simulink model "sim_ballAndPlate"  (R2025a)
settings: Solver=FixedStepAuto  StartTime=0.0  StopTime=inf  FixedStep=0.001  RelTol=1e-3
values from neighbouring files (symbols this model uses):
  a = [xddot; yddot]    [generate_circular_trajectory.m]    (also in generate_square_trajectory.m)
  enable = 1    [setParams.m]
  g = 9.81    [MPC_design.m]    (also in MPC_design_condensed.m; MPC_design_realtime.m; compute_mpc_params.m; setParams.m)
  I_max = 3    [setParams.m]
  inner_I_sat = 1    [setParams.m]
  K_lqr = dlqr(Ad, Bd, Q_lqr, R_lqr)    [setParams.m]
  Km = 11    [setParams.m]
  m = m_a + 1/3 * m_p    (= 0.345333333333)    [setParams.m]
  Q_kf = diag([1, 100, 1, 100])    [setParams.m]
  r = 0.17    [angleToPos.m]    (also in generate_circular_trajectory.m = [x; xdot; y; ydot]; generate_square_trajectory.m = [x; xdot; y; ydot])
  R_kf = diag([0.1, 0.1])    [setParams.m]
  Ts_Inner = 0.001    [setParams.m]
  x0 = sdpvar(nx,1)    [MPC_design.m]    (also in MPC_design_condensed.m = sdpvar(nx, 1); setParams.m = [0, 0, 0, 0])
  x_init = 0    [setParams.m]
  x_max = 0.03    [setParams.m]
undefined symbols (not defined in the file or in its folder): DiscIntNeverNeededParam, G_A, G_B, G_C
libraries: mpclib x1
settings Model: Creator=thoma  LastModifiedBy=thoma

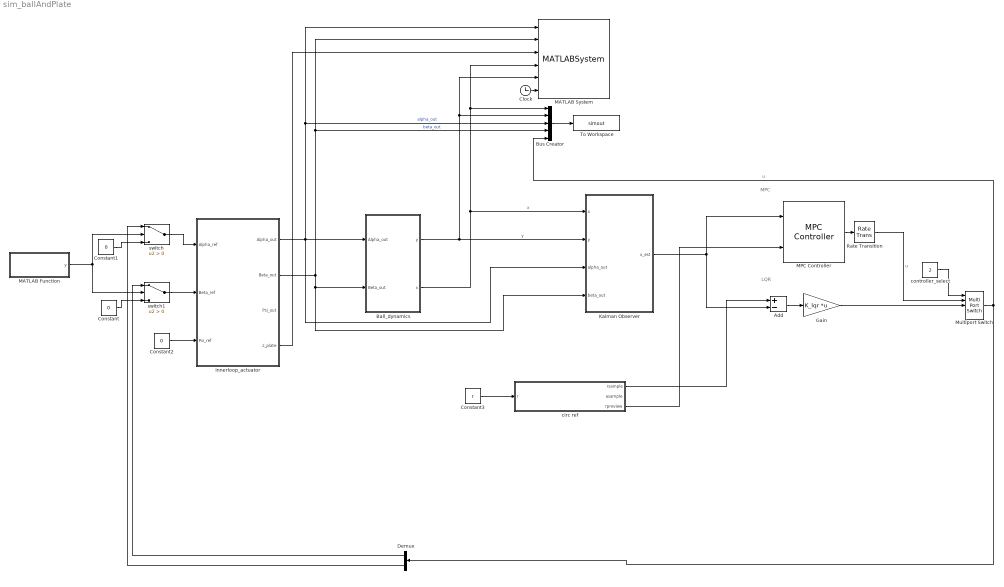
== system sim_ballAndPlate ==
  note: LQR
  note: MPC
  Add : Sum  Inputs=+-
  Ball_dynamics : Subsystem
  Bus Creator : BusCreator  Inputs=5
  Clock : Clock
  Constant : Constant  Value=0
  Constant1 : Constant  Value=0
  Constant2 : Constant  Value=0
  Constant3 : Constant  Value=r
  Demux : Demux  Outputs=2
  Gain : Gain  Gain=K_lqr  Multiplication=Matrix(K*u)
  Innerloop_actuator : Subsystem
  Kalman Observer : Subsystem
  MATLAB Function : MATLAB Function  TreatAsAtomicUnit=on
  MATLAB System : MATLABSystem  System=PlateVisualizer  SimulateUsing=Code generation
      mask Type: PlateVisualizer
  MPC Controller : mpclib/MPC Controller  SCDEnableBlockLinearizationSpecification=on  mpcobj=mpcobj  is_multiple=0  enable_value=0  return_u0=off  updateMPCinCallerWorkspace=on  md_inport=off  mv_inport=off  uref_inport=off  return_cost=off  return_mvseq=off  return_qpstatus=off  return_xseq=off  return_state=off  return_ovseq=off  state_inport=on  umin_inport=off  umax_inport=off  ymin_inport=off  ymax_inport=off  cc_inport=off  ywt_inport=off  uwt_inport=off  duwt_inport=off  rhoeps_inport=off  pm_inport=off  MaximumP=10  HorizonChoice=FixedHorizon  n_ts=0.02  n_p=25  n_mv=2  n_md=0  n_ud=0  n_mo=4  n_uo=0  BlockDataType=double  SampleTimeInherited=off  switch_inport=off
  Multiport Switch : MultiPortSwitch  Inputs=4  SaturateOnIntegerOverflow=off  InputSameDT=off
  Rate Transition : RateTransition
  To Workspace : ToWorkspace  VariableName=simout  SaveFormat=Timeseries  SampleTime=-1
  circ ref : MATLAB Function  TreatAsAtomicUnit=on
  controller_select : Constant  Value=2
  switch : Switch  Criteria=u2 > Threshold  SaturateOnIntegerOverflow=off  InputSameDT=off
  switch1 : Switch  Criteria=u2 > Threshold  SaturateOnIntegerOverflow=off  InputSameDT=off
  wires:
  Constant2/1 -> Innerloop_actuator/3(Psi_ref)
  Innerloop_actuator/2(Beta_out) -> Kalman Observer/4(beta_out), Ball_dynamics/2(Beta_out), Bus Creator/4, MATLAB System/2  "beta_out"
  Innerloop_actuator/1(Alpha_out) -> MATLAB System/1, Bus Creator/3, Kalman Observer/3(alpha_out), Ball_dynamics/1(Alpha_out)  "alpha_out"
  Ball_dynamics/1(y) -> Bus Creator/2, MATLAB System/5, Kalman Observer/2(y)  "y"
  Ball_dynamics/2(x) -> Bus Creator/1, MATLAB System/4, Kalman Observer/1(x)  "x"
  MATLAB Function/1(y) -> switch/2, switch1/2
  Demux/1 -> switch1/1
  switch1/1 -> Innerloop_actuator/2(Beta_ref)
  switch/1 -> Innerloop_actuator/1(Alpha_ref)
  Demux/2 -> switch/1
  Innerloop_actuator/4(z_plate) -> MATLAB System/3
  MPC Controller/1 -> Rate Transition/1
  Multiport Switch/1 -> Demux/1, Bus Creator/5  "u"
  Constant1/1 -> switch/3
  Constant/1 -> switch1/3
  Bus Creator/1 -> To Workspace/1
  Clock/1 -> MATLAB System/6
  circ ref/3(rpreview) -> MPC Controller/2
  Rate Transition/1 -> Multiport Switch/2  "u"
  controller_select/1 -> Multiport Switch/1
  Add/1 -> Gain/1
  circ ref/1(rsample) -> Add/1
  Kalman Observer/1(x_est) -> MPC Controller/1, Add/2
  Gain/1 -> Multiport Switch/3
  Constant3/1 -> circ ref/1(r)

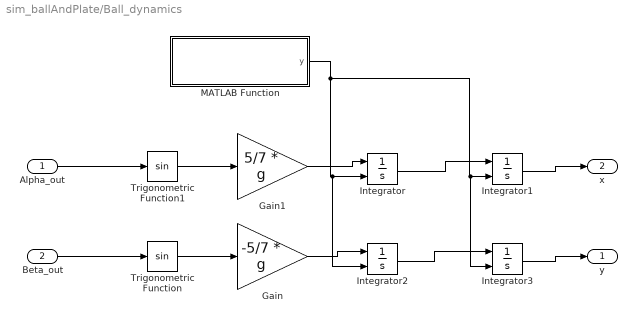
== system sim_ballAndPlate/Ball_dynamics ==
  Alpha_out : Inport
  Beta_out : Inport  Port=2
  Gain : Gain  Gain=-5/7 * g
  Gain1 : Gain  Gain=5/7 * g
  Integrator : Integrator  ExternalReset=rising  InitialCondition=x0(2)
  Integrator1 : Integrator  ExternalReset=rising  InitialCondition=x0(1)
  Integrator2 : Integrator  ExternalReset=rising  InitialCondition=x0(4)
  Integrator3 : Integrator  ExternalReset=rising  InitialCondition=x0(2)
  MATLAB Function : MATLAB Function  TreatAsAtomicUnit=on
  Trigonometric Function : Trigonometry
  Trigonometric Function1 : Trigonometry
  y : Outport
  x : Outport  Port=2
  wires:
  Beta_out/1 -> Trigonometric Function/1
  Trigonometric Function/1 -> Gain/1
  Gain/1 -> Integrator2/1
  Trigonometric Function1/1 -> Gain1/1
  Alpha_out/1 -> Trigonometric Function1/1
  Gain1/1 -> Integrator/1
  Integrator/1 -> Integrator1/1
  Integrator1/1 -> x/1
  Integrator2/1 -> Integrator3/1
  Integrator3/1 -> y/1
  MATLAB Function/1(y) -> Integrator3/2, Integrator1/2, Integrator2/2, Integrator/2

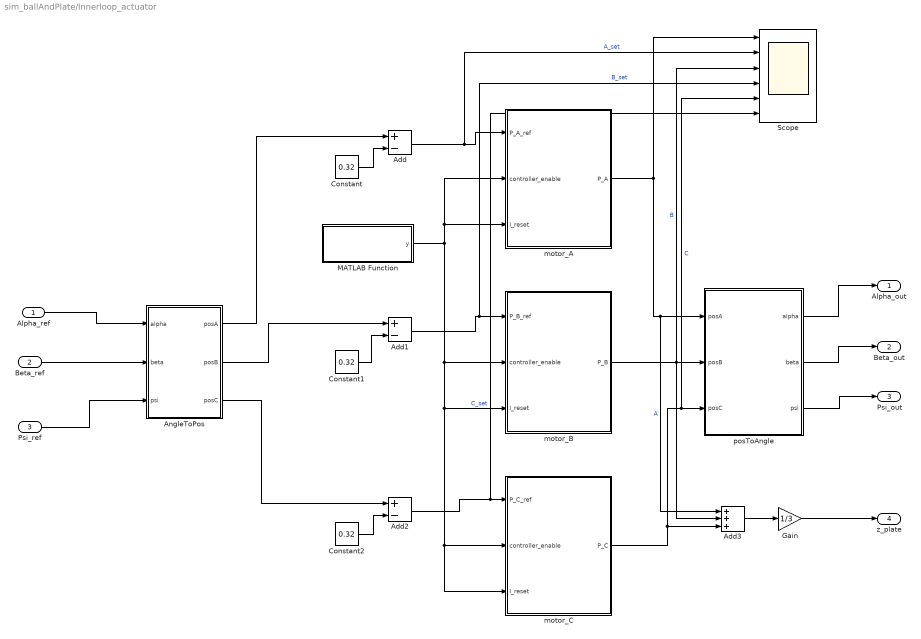
== system sim_ballAndPlate/Innerloop_actuator ==
  Alpha_ref : Inport
  Beta_ref : Inport  Port=2
  Psi_ref : Inport  Port=3
  Add : Sum  Inputs=+-
  Add1 : Sum  Inputs=+-
  Add2 : Sum  Inputs=+-
  Add3 : Sum  Inputs=+++
  "AngleToPos " : MATLAB Function  TreatAsAtomicUnit=on
  Constant : Constant  Value=0.32
  Constant1 : Constant  Value=0.32
  Constant2 : Constant  Value=0.32
  Gain : Gain  Gain=1/3
  MATLAB Function : MATLAB Function  TreatAsAtomicUnit=on
  Scope : Scope  NumInputPorts=6
      settings: ActiveDisplayYMinimum=-0.0017528825710255869  ActiveDisplayYMaximum=0.0020437285369552553
  motor_A : Subsystem
  motor_B : Subsystem
  motor_C : Subsystem
  posToAngle : MATLAB Function  TreatAsAtomicUnit=on
  Alpha_out : Outport
  Beta_out : Outport  Port=2
  Psi_out : Outport  Port=3
  z_plate : Outport  Port=4
  wires:
  Alpha_ref/1 -> "AngleToPos "/1(alpha)
  Beta_ref/1 -> "AngleToPos "/2(beta)
  Psi_ref/1 -> "AngleToPos "/3(psi)
  Constant/1 -> Add/2
  Add/1 -> Scope/2, motor_A/1(P_A_ref)  "A_set"
  motor_A/1(P_A) -> Add3/1, posToAngle/1(posA), Scope/1  "A"
  "AngleToPos "/1(posA) -> Add/1
  posToAngle/1(alpha) -> Alpha_out/1
  "AngleToPos "/2(posB) -> Add1/1
  Add1/1 -> Scope/4, motor_B/1(P_B_ref)  "B_set"
  Constant1/1 -> Add1/2
  "AngleToPos "/3(posC) -> Add2/1
  Add2/1 -> Scope/6, motor_C/1(P_C_ref)  "C_set"
  Constant2/1 -> Add2/2
  motor_C/1(P_C) -> Add3/3, Scope/5, posToAngle/3(posC)  "C"
  motor_B/1(P_B) -> Scope/3, posToAngle/2(posB), Add3/2  "B"
  posToAngle/2(beta) -> Beta_out/1
  posToAngle/3(psi) -> Psi_out/1
  MATLAB Function/1(y) -> motor_B/3(I_reset), motor_C/3(I_reset), motor_C/2(controller_enable), motor_B/2(controller_enable), motor_A/3(I_reset), motor_A/2(controller_enable)
  Add3/1 -> Gain/1
  Gain/1 -> z_plate/1

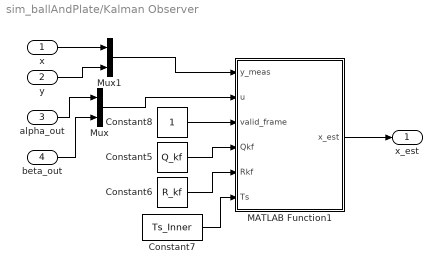
== system sim_ballAndPlate/Kalman Observer ==
  x : Inport
  y : Inport  Port=2
  alpha_out : Inport  Port=3
  beta_out : Inport  Port=4
  Constant5 : Constant  Value=Q_kf
  Constant6 : Constant  Value=R_kf
  Constant7 : Constant  Value=Ts_Inner
  Constant8 : Constant
  MATLAB Function1 : MATLAB Function  TreatAsAtomicUnit=on
  Mux : Mux  Inputs=2
  Mux1 : Mux  Inputs=2
  x_est : Outport
  wires:
  Mux1/1 -> MATLAB Function1/1(y_meas)
  Constant7/1 -> MATLAB Function1/6(Ts)
  Constant5/1 -> MATLAB Function1/4(Qkf)
  x/1 -> Mux1/1
  Mux/1 -> MATLAB Function1/2(u)
  beta_out/1 -> Mux/2
  Constant8/1 -> MATLAB Function1/3(valid_frame)
  Constant6/1 -> MATLAB Function1/5(Rkf)
  MATLAB Function1/1(x_est) -> x_est/1
  y/1 -> Mux1/2
  alpha_out/1 -> Mux/1

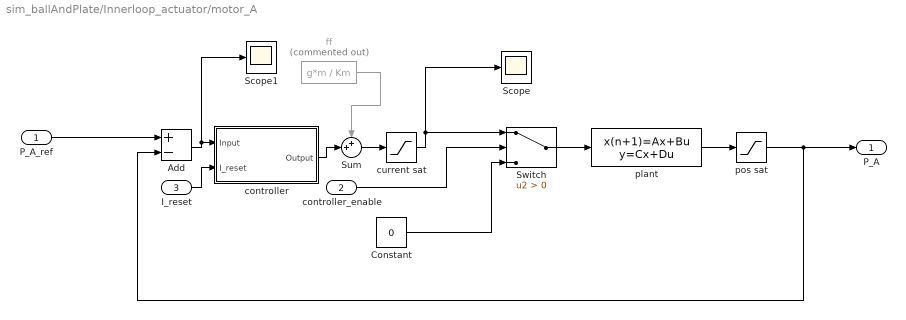
== system sim_ballAndPlate/Innerloop_actuator/motor_A ==
  P_A_ref : Inport
  controller_enable : Inport  Port=2
  I_reset : Inport  Port=3
  Add : Sum  Inputs=+-
  Constant : Constant  Value=0
  Scope : Scope
      settings: ActiveDisplayYMinimum=-0.2151003532733422  ActiveDisplayYMaximum=0.78783772218945147  DataLoggingVariableName=ScopeData3
  Scope1 : Scope
      settings: ActiveDisplayYMinimum=-0.013802200769437761  ActiveDisplayYMaximum=0.022158674956348122  DataLoggingVariableName=ScopeData5
  Sum : Sum  Inputs=++|
  Switch : Switch  Criteria=u2 > Threshold  SaturateOnIntegerOverflow=off  InputSameDT=off
  controller : Subsystem
  current sat : Saturate  UpperLimit=I_max  LowerLimit=-I_max
  ff : Constant  Commented=on  Value=g*m / Km
  plant : DiscreteStateSpace  A=G_A.A  B=G_A.B  C=G_A.C  D=G_A.D  SampleTime=-1
  pos sat : Saturate  UpperLimit=x_max  LowerLimit=-x_max
  P_A : Outport
  wires:
  P_A_ref/1 -> Add/1
  controller/1(Output) -> Sum/2
  plant/1 -> pos sat/1
  pos sat/1 -> Add/2, P_A/1
  controller_enable/1 -> Switch/2
  current sat/1 -> Switch/1, Scope/1
  Switch/1 -> plant/1
  Constant/1 -> Switch/3
  Add/1 -> Scope1/1, controller/1(Input)
  I_reset/1 -> controller/2(I_reset)
  ff/1 -> Sum/1
  Sum/1 -> current sat/1

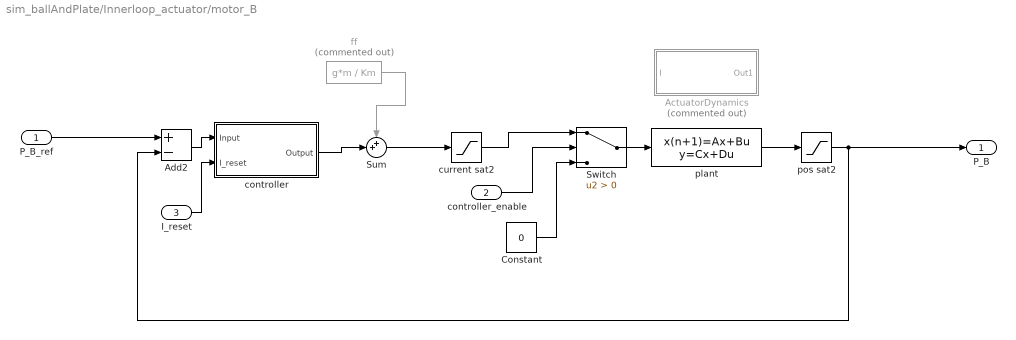
== system sim_ballAndPlate/Innerloop_actuator/motor_B ==
  P_B_ref : Inport
  controller_enable : Inport  Port=2
  I_reset : Inport  Port=3
  ActuatorDynamics : Subsystem  Commented=on
  Add2 : Sum  Inputs=+-
  Constant : Constant  Value=0
  Sum : Sum  Inputs=++|
  Switch : Switch  Criteria=u2 > Threshold  SaturateOnIntegerOverflow=off  InputSameDT=off
  controller : Subsystem
  current sat2 : Saturate  UpperLimit=I_max  LowerLimit=-I_max
  ff : Constant  Commented=on  Value=g*m / Km
  plant : DiscreteStateSpace  A=G_B.A  B=G_B.B  C=G_B.C  D=G_B.D  SampleTime=-1
  pos sat2 : Saturate  UpperLimit=x_max  LowerLimit=-x_max
  P_B : Outport
  wires:
  controller_enable/1 -> Switch/2
  P_B_ref/1 -> Add2/1
  pos sat2/1 -> Add2/2, P_B/1
  Add2/1 -> controller/1(Input)
  controller/1(Output) -> Sum/2
  current sat2/1 -> Switch/1
  Constant/1 -> Switch/3
  ff/1 -> Sum/1
  Sum/1 -> current sat2/1
  Switch/1 -> plant/1
  plant/1 -> pos sat2/1
  I_reset/1 -> controller/2(I_reset)

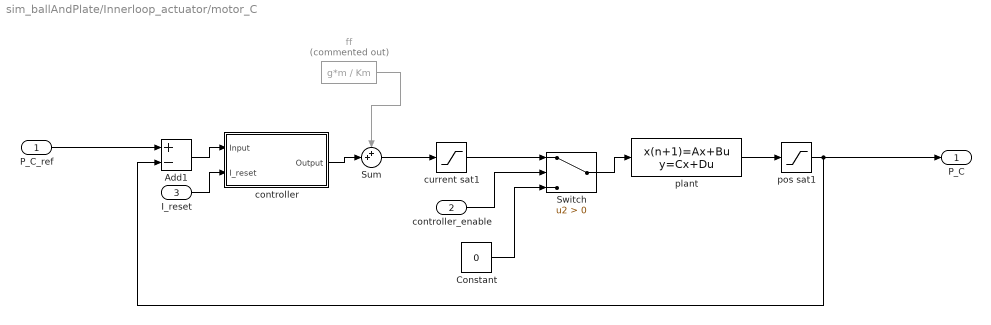
== system sim_ballAndPlate/Innerloop_actuator/motor_C ==
  P_C_ref : Inport
  controller_enable : Inport  Port=2
  I_reset : Inport  Port=3
  Add1 : Sum  Inputs=+-
  Constant : Constant  Value=0
  Sum : Sum  Inputs=++|
  Switch : Switch  Criteria=u2 > Threshold  SaturateOnIntegerOverflow=off  InputSameDT=off
  controller : Subsystem
  current sat1 : Saturate  UpperLimit=I_max  LowerLimit=-I_max
  ff : Constant  Commented=on  Value=g*m / Km
  plant : DiscreteStateSpace  A=G_C.A  B=G_C.B  C=G_C.C  D=G_C.D  SampleTime=-1
  pos sat1 : Saturate  UpperLimit=x_max  LowerLimit=-x_max
  P_C : Outport
  wires:
  controller_enable/1 -> Switch/2
  Switch/1 -> plant/1
  plant/1 -> pos sat1/1
  P_C_ref/1 -> Add1/1
  pos sat1/1 -> Add1/2, P_C/1
  Add1/1 -> controller/1(Input)
  controller/1(Output) -> Sum/2
  current sat1/1 -> Switch/1
  Constant/1 -> Switch/3
  ff/1 -> Sum/1
  Sum/1 -> current sat1/1
  I_reset/1 -> controller/2(I_reset)

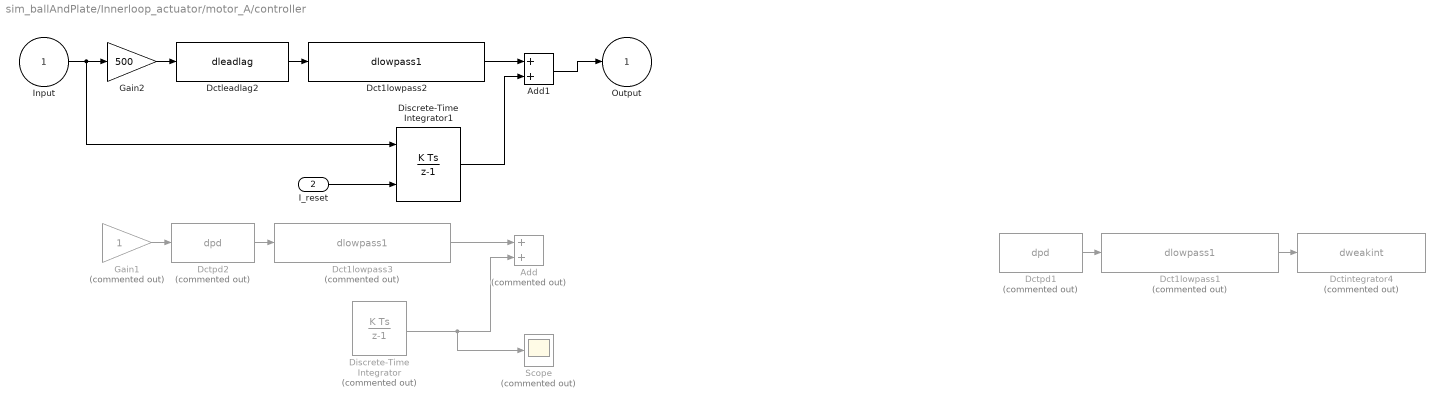
== system sim_ballAndPlate/Innerloop_actuator/motor_A/controller ==
  Input : Inport
  I_reset : Inport  Port=2
  Add : Sum  Commented=on
  Add1 : Sum
  Dct1lowpass1 : S-Function  Commented=on  FunctionName=dlowpass1  Parameters=f_den, 0.001  SFunctionDeploymentMode=off  EnableBusSupport=off  mask(dctools){f_den=200}
      mask prompts: f_den "Pole [Hz]"
      mask help: This block implements a discrete time 1st order lowpass filter.
      mask Display: disp('DCT 1st order lowpass')
  Dct1lowpass2 : S-Function  FunctionName=dlowpass1  Parameters=f_den, 0.001  SFunctionDeploymentMode=off  EnableBusSupport=off  mask(dctools){f_den=50}
      mask prompts: f_den "Pole [Hz]"
      mask help: This block implements a discrete time 1st order lowpass filter.
      mask Display: disp('DCT 1st order lowpass')
  Dct1lowpass3 : S-Function  Commented=on  FunctionName=dlowpass1  Parameters=f_den, 0.001  SFunctionDeploymentMode=off  EnableBusSupport=off  mask(dctools){f_den=200}
      mask prompts: f_den "Pole [Hz]"
      mask help: This block implements a discrete time 1st order lowpass filter.
      mask Display: disp('DCT 1st order lowpass')
  Dctintegrator4 : S-Function  Commented=on  FunctionName=dweakint  Parameters=f_num, 0.001  SFunctionDeploymentMode=off  EnableBusSupport=off  mask(dctools){f_num=1}
      mask prompts: f_num "Zero [Hz]"
      mask help: This block implements a discrete time weak integrator filter.
      mask Display: disp('DCT integrator')
  Dctleadlag2 : S-Function  FunctionName=dleadlag  Parameters=f_num, f_den, 0.001  SFunctionDeploymentMode=off  EnableBusSupport=off  mask(dctools){f_num=7.5, f_den=30}
      mask prompts: f_num "Zero [Hz]"; f_den "Pole [Hz]"
      mask help: This block implements a discrete time leadlag filter.
      mask Display: disp('DCT leadlag')
  Dctpd1 : S-Function  Commented=on  FunctionName=dpd  Parameters=kp, kv, 0.001  SFunctionDeploymentMode=off  EnableBusSupport=off  mask(dctools){kp=0.01, kv=10}
      mask help: This block implements a discrete time pd filter.
      mask Display: disp('DCT pd')
  Dctpd2 : S-Function  Commented=on  FunctionName=dpd  Parameters=kp, kv, 0.001  SFunctionDeploymentMode=off  EnableBusSupport=off  mask(dctools){kp=0.01, kv=10}
      mask help: This block implements a discrete time pd filter.
      mask Display: disp('DCT pd')
  Discrete-Time Integrator : DiscreteIntegrator  Commented=on  gainval=1  ExternalReset=rising  SampleTime=-1  ICPrevOutput=DiscIntNeverNeededParam  ICPrevScaledInput=DiscIntNeverNeededParam
  Discrete-Time Integrator1 : DiscreteIntegrator  gainval=3531  ExternalReset=rising  SampleTime=-1  LimitOutput=on  UpperSaturationLimit=inner_I_sat  LowerSaturationLimit=-inner_I_sat  ICPrevOutput=DiscIntNeverNeededParam  ICPrevScaledInput=DiscIntNeverNeededParam
  Gain1 : Gain  Commented=on
  Gain2 : Gain  Gain=500  SaturateOnIntegerOverflow=on  OutDataTypeStr=Inherit: Same as input  ParamDataTypeStr=Inherit: Same as input
  Scope : Scope  Commented=on
      settings: ActiveDisplayYMinimum=-6.500387462094743E-17  ActiveDisplayYMaximum=0  DataLoggingVariableName=ScopeData8
  Output : Outport
  wires:
  Gain1/1 -> Dctpd2/1
  Dctpd2/1 -> Dct1lowpass3/1
  Dct1lowpass3/1 -> Add/1
  Discrete-Time Integrator/1 -> Scope/1, Add/2
  Dctpd1/1 -> Dct1lowpass1/1
  Dct1lowpass1/1 -> Dctintegrator4/1
  Input/1 -> Discrete-Time Integrator1/1, Gain2/1
  Discrete-Time Integrator1/1 -> Add1/2
  I_reset/1 -> Discrete-Time Integrator1/2
  Gain2/1 -> Dctleadlag2/1
  Dct1lowpass2/1 -> Add1/1
  Dctleadlag2/1 -> Dct1lowpass2/1
  Add1/1 -> Output/1

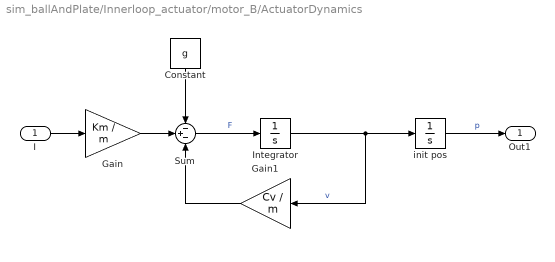
== system sim_ballAndPlate/Innerloop_actuator/motor_B/ActuatorDynamics ==
  I : Inport
  Constant : Constant  Value=g
  Gain : Gain  Gain=Km / m
  Gain1 : Gain  Gain=Cv / m
  Integrator : Integrator
  Sum : Sum  Inputs=-+-
  init pos : Integrator  InitialCondition=x_init
  Out1 : Outport
  wires:
  I/1 -> Gain/1
  Gain/1 -> Sum/2
  init pos/1 -> Out1/1  "p"
  Sum/1 -> Integrator/1  "F"
  Integrator/1 -> Gain1/1, init pos/1  "v"
  Gain1/1 -> Sum/3
  Constant/1 -> Sum/1

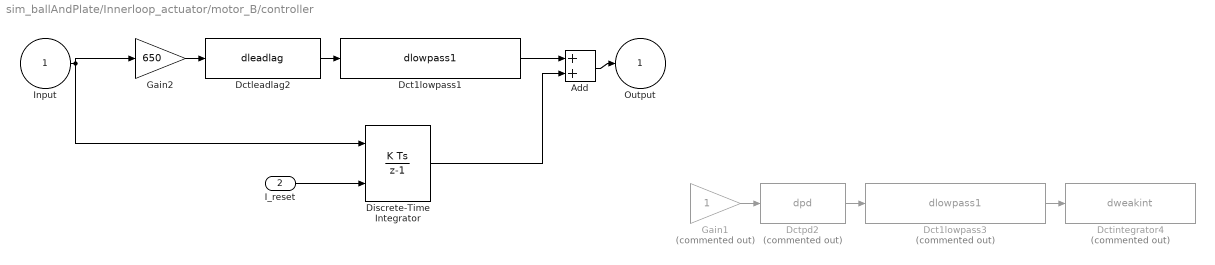
== system sim_ballAndPlate/Innerloop_actuator/motor_B/controller ==
  Input : Inport
  I_reset : Inport  Port=2
  Add : Sum
  Dct1lowpass1 : S-Function  FunctionName=dlowpass1  Parameters=f_den, 0.001  SFunctionDeploymentMode=off  EnableBusSupport=off  mask(dctools){f_den=50}
      mask prompts: f_den "Pole [Hz]"
      mask help: This block implements a discrete time 1st order lowpass filter.
      mask Display: disp('DCT 1st order lowpass')
  Dct1lowpass3 : S-Function  Commented=on  FunctionName=dlowpass1  Parameters=f_den, 0.001  SFunctionDeploymentMode=off  EnableBusSupport=off  mask(dctools){f_den=200}
      mask prompts: f_den "Pole [Hz]"
      mask help: This block implements a discrete time 1st order lowpass filter.
      mask Display: disp('DCT 1st order lowpass')
  Dctintegrator4 : S-Function  Commented=on  FunctionName=dweakint  Parameters=f_num, 0.001  SFunctionDeploymentMode=off  EnableBusSupport=off  mask(dctools){f_num=1}
      mask prompts: f_num "Zero [Hz]"
      mask help: This block implements a discrete time weak integrator filter.
      mask Display: disp('DCT integrator')
  Dctleadlag2 : S-Function  FunctionName=dleadlag  Parameters=f_num, f_den, 0.001  SFunctionDeploymentMode=off  EnableBusSupport=off  mask(dctools){f_num=7.5, f_den=30}
      mask prompts: f_num "Zero [Hz]"; f_den "Pole [Hz]"
      mask help: This block implements a discrete time leadlag filter.
      mask Display: disp('DCT leadlag')
  Dctpd2 : S-Function  Commented=on  FunctionName=dpd  Parameters=kp, kv, 0.001  SFunctionDeploymentMode=off  EnableBusSupport=off  mask(dctools){kp=0.01, kv=10}
      mask help: This block implements a discrete time pd filter.
      mask Display: disp('DCT pd')
  Discrete-Time Integrator : DiscreteIntegrator  gainval=4102  ExternalReset=rising  SampleTime=-1  LimitOutput=on  UpperSaturationLimit=inner_I_sat  LowerSaturationLimit=-inner_I_sat  ICPrevOutput=DiscIntNeverNeededParam  ICPrevScaledInput=DiscIntNeverNeededParam
  Gain1 : Gain  Commented=on
  Gain2 : Gain  Gain=650  SaturateOnIntegerOverflow=on  OutDataTypeStr=Inherit: Same as input  ParamDataTypeStr=Inherit: Same as input
  Output : Outport
  wires:
  Gain1/1 -> Dctpd2/1
  Dctpd2/1 -> Dct1lowpass3/1
  Dct1lowpass3/1 -> Dctintegrator4/1
  Input/1 -> Gain2/1, Discrete-Time Integrator/1
  I_reset/1 -> Discrete-Time Integrator/2
  Discrete-Time Integrator/1 -> Add/2
  Dct1lowpass1/1 -> Add/1
  Gain2/1 -> Dctleadlag2/1
  Dctleadlag2/1 -> Dct1lowpass1/1
  Add/1 -> Output/1

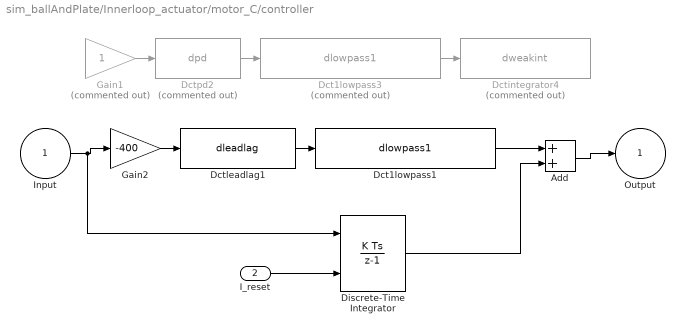
== system sim_ballAndPlate/Innerloop_actuator/motor_C/controller ==
  Input : Inport
  I_reset : Inport  Port=2
  Add : Sum
  Dct1lowpass1 : S-Function  FunctionName=dlowpass1  Parameters=f_den, 0.001  SFunctionDeploymentMode=off  EnableBusSupport=off  mask(dctools){f_den=50}
      mask prompts: f_den "Pole [Hz]"
      mask help: This block implements a discrete time 1st order lowpass filter.
      mask Display: disp('DCT 1st order lowpass')
  Dct1lowpass3 : S-Function  Commented=on  FunctionName=dlowpass1  Parameters=f_den, 0.001  SFunctionDeploymentMode=off  EnableBusSupport=off  mask(dctools){f_den=200}
      mask prompts: f_den "Pole [Hz]"
      mask help: This block implements a discrete time 1st order lowpass filter.
      mask Display: disp('DCT 1st order lowpass')
  Dctintegrator4 : S-Function  Commented=on  FunctionName=dweakint  Parameters=f_num, 0.001  SFunctionDeploymentMode=off  EnableBusSupport=off  mask(dctools){f_num=1}
      mask prompts: f_num "Zero [Hz]"
      mask help: This block implements a discrete time weak integrator filter.
      mask Display: disp('DCT integrator')
  Dctleadlag1 : S-Function  FunctionName=dleadlag  Parameters=f_num, f_den, 0.001  SFunctionDeploymentMode=off  EnableBusSupport=off  mask(dctools){f_num=7.5, f_den=30}
      mask prompts: f_num "Zero [Hz]"; f_den "Pole [Hz]"
      mask help: This block implements a discrete time leadlag filter.
      mask Display: disp('DCT leadlag')
  Dctpd2 : S-Function  Commented=on  FunctionName=dpd  Parameters=kp, kv, 0.001  SFunctionDeploymentMode=off  EnableBusSupport=off  mask(dctools){kp=0.01, kv=10}
      mask help: This block implements a discrete time pd filter.
      mask Display: disp('DCT pd')
  Discrete-Time Integrator : DiscreteIntegrator  gainval=2500  ExternalReset=rising  SampleTime=-1  LimitOutput=on  UpperSaturationLimit=inner_I_sat  LowerSaturationLimit=-inner_I_sat  ICPrevOutput=DiscIntNeverNeededParam  ICPrevScaledInput=DiscIntNeverNeededParam
  Gain1 : Gain  Commented=on
  Gain2 : Gain  Gain=-400  SaturateOnIntegerOverflow=on  OutDataTypeStr=Inherit: Same as input  ParamDataTypeStr=Inherit: Same as input
  Output : Outport
  wires:
  Gain1/1 -> Dctpd2/1
  Dctpd2/1 -> Dct1lowpass3/1
  Dct1lowpass3/1 -> Dctintegrator4/1
  Gain2/1 -> Dctleadlag1/1
  Input/1 -> Discrete-Time Integrator/1, Gain2/1
  I_reset/1 -> Discrete-Time Integrator/2
  Dct1lowpass1/1 -> Add/1
  Discrete-Time Integrator/1 -> Add/2
  Dctleadlag1/1 -> Dct1lowpass1/1
  Add/1 -> Output/1

== matlab function sim_ballAndPlate/MATLAB Function ==
  data: y output
function y = get_outer_loop_state()
    % This block queries the base workspace live at every single sample step
    % We declare evalin as extrinsic so the code generator bypasses it
    coder.extrinsic('evalin');
    
    % Initialize a safe compiled default value
    state_val = 0.0; 
    
    % Safely read the value from the MATLAB base workspace
    state_val = evalin('base', 'outer_loop_enable');
    
    % Cast the value to a standard double output
    y = double(state_val);
end

== matlab function sim_ballAndPlate/Innerloop_actuator/posToAngle ==
  data: posA input; alpha output; posB input; posC input; beta output; psi output
function [alpha, beta, psi] = posToAngle(posA, posB, posC)
    % Returns the angles resulting from the given position
    % note: the position should be relative from the actuators midpoint in the global frame

    % Physical Constants
    r = 0.17;                 % Radius to joints (m)
    h = 0.322;                % Resting height (m)
    theta = deg2rad(120);     % angle between bases (rad)

    % Reconstruction of the Plate Unit Vectors 
    % We find where the joints are in the world frame by using the inputs
    % If pos = 0.322, the joints are exactly T_height above the base.
    P1_global = [r; 0; h + posA];
    P2_global = [r*cos(theta); r*sin(theta); h + posB];
    P3_global = [r*cos(theta); -r*sin(theta); h + posC];

    % Find the center of the tilted plate
    % The average of the three joint positions gives the center of the motion plate
    center = (P1_global + P2_global + P3_global) / 3;

    % Vectors from the plate center to the joints
    % This isolates the tilt of the plate surface
    v1 = P1_global - center;
    v2 = P2_global - center;
    v3 = P3_global - center;

    % Compute Unit Vectors
    uX = v1 / norm(v1);             % Plate X-axis
    u_temp = cross(uX, v3);         % Temporary vector to find normal
    uZ = u_temp / norm(u_temp);     % Plate Z-axis (Normal)
    uY = cross(uZ, uX);             % Plate Y-axis

    % Extract Tait-Bryan Angles
    beta = asin(-uX(3));                            
    alpha = asin(uY(3) / sqrt(1 - uX(3)^2));       
    psi = asin(uX(2) / sqrt(1 - uX(3)^2));
end

== matlab function sim_ballAndPlate/Innerloop_actuator/MATLAB Function ==
  data: y output
function y = get_inner_loop_state()
    % This block queries the base workspace live at every single sample step
    % We declare evalin as extrinsic so the code generator bypasses it
    coder.extrinsic('evalin');
    
    % Initialize a safe compiled default value
    state_val = 0.0; 
    
    % Safely read the value from the MATLAB base workspace
    state_val = evalin('base', 'inner_loop_enable');
    
    % Cast the value to a standard double output
    y = double(state_val);
end

== matlab function sim_ballAndPlate/Ball_dynamics/MATLAB Function ==
  data: y output
function y = get_sim_reset_loop_state()
    % This block queries the base workspace live at every single sample step
    % We declare evalin as extrinsic so the code generator bypasses it
    coder.extrinsic('evalin');
    
    % Initialize a safe compiled default value
    state_val = 0.0; 
    
    % Safely read the value from the MATLAB base workspace
    state_val = evalin('base', 'sim_reset');
    
    % Cast the value to a standard double output
    y = double(state_val);
end

== matlab function sim_ballAndPlate/Innerloop_actuator/AngleToPos  ==
  data: alpha input; posA output; beta input; psi input; posB output; posC output
function [posA, posB, posC] = angleToPos(alpha, beta, psi)
    % Returns the actuator positions required to reach the desired angle
    % note: the position is absolute in the global frame

    % Physical Constants
    r = 0.17;           % Joint radius (m)
    h = [0; 0; 0.32];  % Resting height vector (m)
    
    % Joint positions on base and plate (equilateral triangle)
    % These match the definitions in your posToAngle function
    theta = [0, deg2rad(240), deg2rad(120)];
    B = [r*cos(theta); r*sin(theta); zeros(1,3)]; % Base joints (b_i)
    P = [r*cos(theta); r*sin(theta); zeros(1,3)]; % Plate joints (p_i)
    
    % Rotation Matrices (Yaw-Pitch-Roll order)
    Rz = [cos(psi) -sin(psi) 0; sin(psi) cos(psi) 0; 0 0 1];
    Ry = [cos(beta) 0 sin(beta); 0 1 0; -sin(beta) 0 cos(beta)];
    Rx = [1 0 0; 0 cos(alpha) -sin(alpha); 0 sin(alpha) cos(alpha)];
    R_BtoP = Rz * Ry * Rx; 
    
    % Compute absolute position for each motor
    % Motor 1
    l1_vec = h + (R_BtoP * P(:,1)) - B(:,1);
    posA = norm(l1_vec);
    
    % Motor 2
    l2_vec = h + (R_BtoP * P(:,2)) - B(:,2);
    posB = norm(l2_vec);
    
    % Motor 3
    l3_vec = h + (R_BtoP * P(:,3)) - B(:,3);
    posC = norm(l3_vec);
end

== matlab function sim_ballAndPlate/Kalman Observer/MATLAB Function1 ==
  settings: updateMethod=DISCRETE
  data: y_meas input; u input; x_est output; valid_frame input; Qkf input; Rkf input; Ts input
function x_est = intermittent_kalman(y_meas, u, valid_frame, Qkf, Rkf, Ts)
    
    g = 9.81;
    Ad = [1, Ts, 0,0;
        0, 1, 0, 0;
        0, 0, 1, Ts;
        0, 0, 0, 1];

    Bd = [5/14 * g * Ts^2, 0;
        5/7 * g * Ts, 0;
        0, 5/14 * g * Ts^2;
        0, 5/7 * g * Ts];
    
    Cd = [1 0 0 0;
        0 0 1 0];


    % Persistent variables keep their state between sample steps
    persistent x_hat P
    
    % Initialization on the very first time step
    if isempty(x_hat)
        x_hat = zeros(4,1);
        P = eye(4) * 0.1;
    end
    
    % 1. Prediction Step (Always executes)
    x_pred = Ad * x_hat + Bd * u;
    P_pred = Ad * P * Ad' + Qkf;
    
    % 2. Correction Step (Conditional)
    if valid_frame > 0.5
        % Frame is valid: Run normal Kalman Correction
        S = Cd * P_pred * Cd' + Rkf;
        K = P_pred * Cd' / S; % Equivalent to P_pred * Cd' * inv(S)
        
        x_hat = x_pred + K * (y_meas - Cd * x_pred);
        lastxhatvalid = x_hat;
        P = (eye(4) - K * Cd) * P_pred;
    else
        % Frame was dropped: Skip correction, trust physics prediction
        x_hat = x_hat;
        P = P_pred;
    end
    
    % Output the current state estimate
    x_est = x_hat;
end

== matlab function sim_ballAndPlate/circ ref ==
  data: r input double; rsample output double size=[4,1]; asample output double size=[2,1]; a parameter double; enable parameter double; rpreview output double size=[25, 4]
function [rsample, asample, rpreview] = ref_player(r, a, enable)
%#codegen
Npreview = 25; % number of samples preview for MPC

% Persistent variable to track the current sample index
persistent idx_ref;

% Initialize the index on the very first time step
if isempty(idx_ref)
    idx_ref = 1;
end

% Determine the total number of offline samples available
N_total = size(r, 2);

% Preallocate outputs for code generation stability
rsample = zeros(4, 1);
asample = zeros(2, 1);
% CHANGED: 25 rows (time steps), 4 columns (states)
rpreview = zeros(Npreview, 4); 

% --- Trajectory Generation Logic ---
if enable == 1
    % 1. Extract the current sample
    if idx_ref <= N_total
        rsample = r(:, idx_ref);
        asample = a(:, idx_ref);
    else
        % Hold the final sample if the trajectory ends but enable stays 1
        rsample = r(:, N_total);
        asample = a(:, N_total);
    end
    
    % 2. Extract the next Npreview samples for MPC
    for i = 1:Npreview
        preview_idx = idx_ref + i; 
        
        if preview_idx <= N_total
            % CHANGED: Assign transposed column [1x4] into row i
            rpreview(i, :) = r(:, preview_idx)'; 
        else
            % Zero-order hold: Pad with the last available reference state 
            rpreview(i, :) = r(:, N_total)';
        end
    end
    
    % 3. Advance the index for the next sample time (Ts)
    if idx_ref <= N_total
        idx_ref = idx_ref + 1;
    end
else
    % --- Reset / Idle State (enable == 0) ---
    % Keep index reset to the first sample
    idx_ref = 1; 
    
    % Output the initial conditions while waiting
    rsample = r(:, 1);
    asample = a(:, 1);
    
    % Provide a static look-ahead from the starting point
    for i = 1:Npreview
        if (1 + i) <= N_total
            % CHANGED: Transpose required here too
            rpreview(i, :) = r(:, 1 + i)';
        else
            rpreview(i, :) = r(:, N_total)';
        end
    end
end
